simulink model "BMS_OL_Harness_advancedcell"  (R2017b)
settings: Solver=FixedStepDiscrete  StartTime=0.0  StopTime=660  FixedStep=BMSk_stepSize  RelTol=1e-3  EnableMultiTasking=on
values from neighbouring files (symbols this model uses):
  BMSk_stepSize = 0.1    [BMS_OL_init.m]
settings Model: PauseTimes=22  Creator=ms2zwt  LastModifiedBy=nctzv8
settings ConfigSet: Description=OpenECU configuration set for code generation under RTW-EC.
settings SolverCC: PositivePriorityOrder=on
settings DataIOCC: LimitDataPoints=on  SaveFormat=Array  SignalLoggingSaveFormat=ModelDataLogs
settings OptimizationCC: DefaultParameterBehavior=Inlined  InlineInvariantSignals=on  ExpressionDepthLimit=2147483647  StateBitsets=on  DataBitsets=on  ZeroExternalMemoryAtStartup=off  ZeroInternalMemoryAtStartup=off  NoFixptDivByZeroProtection=on  EfficientFloat2IntCast=on  LifeSpan=1
settings DebuggingCC: SaveWithParameterizedLinksMsg=none  UnderspecifiedInitializationDetection=Classic  MergeDetectMultiDrivingBlocksExec=none  SignalResolutionControl=TryResolveAllWithWarning  MultiTaskDSMMsg=warning  MultiTaskCondExecSysMsg=none  SingleTaskRateTransMsg=error  CheckMatrixSingularityMsg=warning  VectorMatrixConversionMsg=warning  FcnCallInpInsideContextMsg=warning  SignalLabelMismatchMsg=warning  AllowSymbolicDim=off  StateNameClashWarn=warning  SFUnexpectedBacktrackingDiag=warning  SFNoUnconditionalDefaultTransitionDiag=warning  SFExecutionAtInitializationDiag=none
settings HardwareCC: ProdBitPerPointer=32  ProdBitPerSizeT=32  ProdBitPerPtrDiffT=32  ProdLargestAtomicInteger=Long  ProdLargestAtomicFloat=Double  ProdEndianess=BigEndian  ProdWordSize=32  ProdHWDeviceType=Freescale->32-bit PowerPC  TargetIntDivRoundTo=Zero  TargetEndianess=BigEndian  TargetHWDeviceType=Freescale->32-bit PowerPC  ProdEqTarget=off
settings ModelReferenceCC: PropagateSignalLabelsOutOfModel=off
settings SFSimCC: MATLABDynamicMemAlloc=off
settings RTWCC: SystemTargetFile=openecu_ert.tlc  MakeCommand=make_rtw optimized_floating_point=1  TemplateMakefile=openecu_ert_r2015b_64.tmf  Description=OpenECU Platform Target (ERT, optimised floating-point code)  RetainRTWFile=on  IncludeHyperlinkInReport=on
settings CodeAppCC: ForceParamTrailComments=on  IgnoreCustomStorageClasses=off  SimulinkDataObjDesc=on  CustomSymbolStrType=$N$R$M  InsertBlockDesc=on  StateflowObjectComments=on  InternalIdentifier=Classic
settings STFCustomTargetCC: TargetLibSuffix=.a  GenerateSampleERTMain=on  IncludeMdlTerminateFcn=off  CombineOutputUpdateFcns=on  IncludeFileDelimiter=UseQuote  ERTCustomFileBanners=on  SupportContinuousTime=off  RemoveResetFunc=on  MATLABClassNameForMDSCustomization=Simulink.SoftwareTarget.ERTCustomization  GRTInterface=off  SystemTargetFile=openecu_ert.tlc
settings ERTTargetCC: MultiwordLength=2048  GenerateSampleERTMain=on  ParMdlRefBuildCompliant=off  CompOptLevelCompliant=off  ConcurrentExecutionCompliant=off  IncludeMdlTerminateFcn=off  IncludeFileDelimiter=UseQuote  SupportNonInlinedSFcns=on  ModelStepFunctionPrototypeControlCompliant=off  CPPClassGenCompliant=off  UseToolchainInfoCompliant=off  ExtModeMexFile=noextcomm  InlinedParameterPlacement=NonHierarchical  ERTSrcFileBannerTemplate=oe_code_c_template.cgt  ERTHdrFileBannerTemplate=oe_code_h_template.cgt  ERTDataSrcFileTemplate=oe_data_c_template.cgt  ERTDataHdrFileTemplate=oe_data_h_template.cgt  ERTCustomFileTemplate=example_file_process.tlc  GlobalDataDefinition=InSeparateSourceFile  GlobalDataReference=InSeparateHeaderFile  ConvertIfToSwitch=off  SuppressUnreachableDefaultCases=off  EnableUserReplacementTypes=on
settings ConfigComp: CovMetricSettings=dw  CovHtmlReporting=on  CovSaveCumulativeToWorkspaceVar=on  CovSaveSingleToWorkspaceVar=on  CovExternalEMLEnable=off

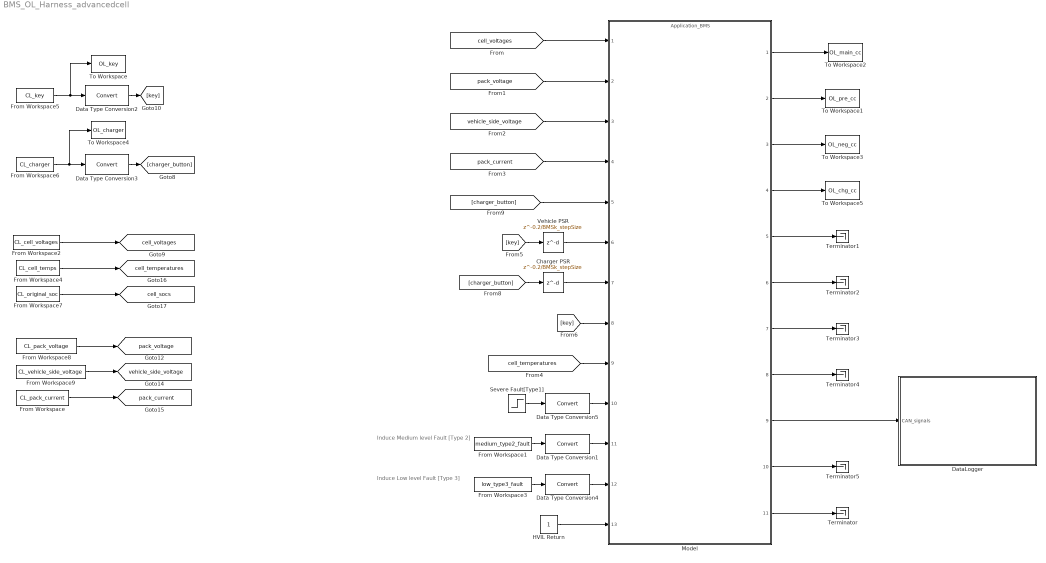
== system BMS_OL_Harness_advancedcell ==
  note: Induce Medium level Fault
      | [Type 2]
  note: Induce Low level Fault
      | [Type 3]
  Charger PSR : Delay  DelayLength=0.2/BMSk_stepSize
  Data Type Conversion{1..5} (5 alike) : DataTypeConversion
  DataLogger : Subsystem
  From Workspace : FromWorkspace  VariableName=CL_pack_current  SampleTime=BMSk_stepSize
  From Workspace1 : FromWorkspace  VariableName=medium_type2_fault  SampleTime=BMSk_stepSize
  From Workspace2 : FromWorkspace  VariableName=CL_cell_voltages  SampleTime=BMSk_stepSize
  From Workspace3 : FromWorkspace  VariableName=low_type3_fault  SampleTime=BMSk_stepSize
  From Workspace4 : FromWorkspace  VariableName=CL_cell_temps  SampleTime=BMSk_stepSize
  From Workspace5 : FromWorkspace  VariableName=CL_key  SampleTime=BMSk_stepSize
  From Workspace6 : FromWorkspace  VariableName=CL_charger  SampleTime=BMSk_stepSize
  From Workspace7 : FromWorkspace  VariableName=CL_original_soc  SampleTime=BMSk_stepSize
  From Workspace8 : FromWorkspace  VariableName=CL_pack_voltage  SampleTime=BMSk_stepSize
  From Workspace9 : FromWorkspace  VariableName=CL_vehicle_side_voltage  SampleTime=BMSk_stepSize
  HVIL Return : Constant  OutDataTypeStr=double  SampleTime=-1
  Model : ModelReference  ModelNameDialog=Application_BMS.slx  SimulationMode=Normal  ModelReferenceVersion=1.801
  Severe Fault[Type1] : Step  Time=0  After=0
  Terminator{,1..5} (6 alike) : Terminator
  To Workspace : ToWorkspace  VariableName=OL_key  SaveFormat=Timeseries  SampleTime=-1
  To Workspace1 : ToWorkspace  VariableName=OL_pre_cc  SaveFormat=Timeseries  SampleTime=-1
  To Workspace2 : ToWorkspace  VariableName=OL_main_cc  SaveFormat=Timeseries  SampleTime=-1
  To Workspace3 : ToWorkspace  VariableName=OL_neg_cc  SaveFormat=Timeseries  SampleTime=-1
  To Workspace4 : ToWorkspace  VariableName=OL_charger  SaveFormat=Timeseries  SampleTime=-1
  To Workspace5 : ToWorkspace  VariableName=OL_chg_cc  SaveFormat=Timeseries  SampleTime=-1
  Vehicle PSR : Delay  DelayLength=0.2/BMSk_stepSize
  tag scope: cell_socs=global, cell_temperatures=global, cell_voltages=global, pack_current=global, pack_voltage=global, vehicle_side_voltage=global
  wires:
  [cell_temperatures] -> Model/9
  Vehicle PSR/1 -> Model/6
  [key] -> Vehicle PSR/1
  [key] -> Model/8
  [charger_button] -> Model/5
  Charger PSR/1 -> Model/7
  [charger_button] -> Charger PSR/1
  Model/4 -> To Workspace5/1
  Model/3 -> To Workspace3/1
  Model/1 -> To Workspace2/1
  Data Type Conversion2/1 -> [key]
  Data Type Conversion4/1 -> Model/12
  From Workspace1/1 -> Data Type Conversion1/1
  Data Type Conversion5/1 -> Model/10
  [pack_current] -> Model/4
  [vehicle_side_voltage] -> Model/3
  [pack_voltage] -> Model/2
  [cell_voltages] -> Model/1
  Model/9 -> DataLogger/1(CAN_signals)
  Model/2 -> To Workspace1/1
  Data Type Conversion3/1 -> [charger_button]
  From Workspace5/1 -> To Workspace/1, Data Type Conversion2/1
  From Workspace6/1 -> To Workspace4/1, Data Type Conversion3/1
  Data Type Conversion1/1 -> Model/11
  Model/11 -> Terminator/1
  HVIL Return/1 -> Model/13
  From Workspace3/1 -> Data Type Conversion4/1
  Model/5 -> Terminator1/1
  Model/6 -> Terminator2/1
  Model/7 -> Terminator3/1
  Model/8 -> Terminator4/1
  Model/10 -> Terminator5/1
  From Workspace2/1 -> [cell_voltages]
  From Workspace4/1 -> [cell_temperatures]
  From Workspace7/1 -> [cell_socs]
  From Workspace8/1 -> [pack_voltage]
  From Workspace9/1 -> [vehicle_side_voltage]
  From Workspace/1 -> [pack_current]
  Severe Fault[Type1]/1 -> Data Type Conversion5/1

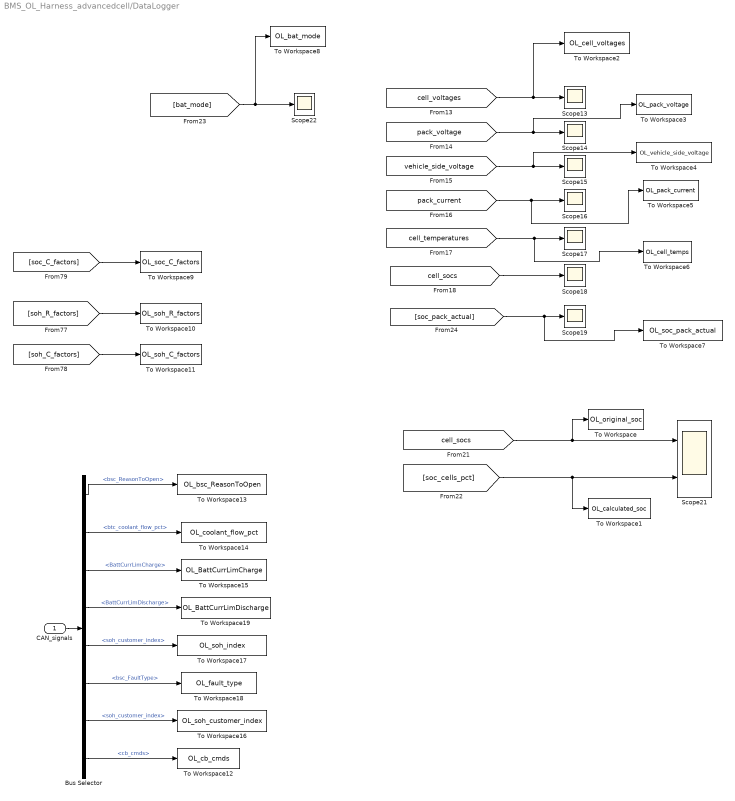
== system BMS_OL_Harness_advancedcell/DataLogger ==
  CAN_signals : Inport
  Bus Selector : BusSelector  OutputSignals=bsc_output.bsc_ReasonToOpen,btc_output.btc_coolant_flow_pct,sop_output.BattCurrLimCharge,sop_output.BattCurrLimDischarge,soh_output.soh_customer_index,bsc_output.bsc_FaultType,soh_output.soh_customer_index,cb_output.cb_cmds
  Scope{13..19,22} (8 alike) : Scope
  Scope21 : Scope  NumInputPorts=2
  To Workspace : ToWorkspace  VariableName=OL_original_soc  SaveFormat=Timeseries  SampleTime=-1
  To Workspace1 : ToWorkspace  VariableName=OL_calculated_soc  SaveFormat=Timeseries  SampleTime=-1
  To Workspace10 : ToWorkspace  VariableName=OL_soh_R_factors  SaveFormat=Timeseries  SampleTime=-1
  To Workspace11 : ToWorkspace  VariableName=OL_soh_C_factors  SaveFormat=Timeseries  SampleTime=-1
  To Workspace12 : ToWorkspace  VariableName=OL_cb_cmds  SaveFormat=Timeseries  SampleTime=-1
  To Workspace13 : ToWorkspace  VariableName=OL_bsc_ReasonToOpen  SaveFormat=Timeseries  SampleTime=-1
  To Workspace14 : ToWorkspace  VariableName=OL_coolant_flow_pct  SaveFormat=Timeseries  SampleTime=-1
  To Workspace15 : ToWorkspace  VariableName=OL_BattCurrLimCharge  SaveFormat=Timeseries  SampleTime=-1
  To Workspace16 : ToWorkspace  VariableName=OL_soh_customer_index  SaveFormat=Timeseries  SampleTime=-1
  To Workspace17 : ToWorkspace  VariableName=OL_soh_index  SaveFormat=Timeseries  SampleTime=-1
  To Workspace18 : ToWorkspace  VariableName=OL_fault_type  SaveFormat=Timeseries  SampleTime=-1
  To Workspace19 : ToWorkspace  VariableName=OL_BattCurrLimDischarge  SaveFormat=Timeseries  SampleTime=-1
  To Workspace2 : ToWorkspace  VariableName=OL_cell_voltages  SaveFormat=Timeseries  SampleTime=-1
  To Workspace3 : ToWorkspace  VariableName=OL_pack_voltage  SaveFormat=Timeseries  SampleTime=-1
  To Workspace4 : ToWorkspace  VariableName=OL_vehicle_side_voltage  SaveFormat=Timeseries  SampleTime=-1
  To Workspace5 : ToWorkspace  VariableName=OL_pack_current  SaveFormat=Timeseries  SampleTime=-1
  To Workspace6 : ToWorkspace  VariableName=OL_cell_temps  SaveFormat=Timeseries  SampleTime=-1
  To Workspace7 : ToWorkspace  VariableName=OL_soc_pack_actual  SaveFormat=Timeseries  SampleTime=-1
  To Workspace8 : ToWorkspace  VariableName=OL_bat_mode  SaveFormat=Timeseries  SampleTime=-1
  To Workspace9 : ToWorkspace  VariableName=OL_soc_C_factors  SaveFormat=Timeseries  SampleTime=-1
  wires:
  [cell_voltages] -> To Workspace2/1, Scope13/1
  [pack_voltage] -> To Workspace3/1, Scope14/1
  [vehicle_side_voltage] -> To Workspace4/1, Scope15/1
  [pack_current] -> To Workspace5/1, Scope16/1
  [cell_temperatures] -> To Workspace6/1, Scope17/1
  [cell_socs] -> Scope18/1
  [cell_socs] -> To Workspace/1, Scope21/1
  [bat_mode] -> To Workspace8/1, Scope22/1
  [soc_cells_pct] -> To Workspace1/1, Scope21/2
  [soc_pack_actual] -> To Workspace7/1, Scope19/1
  [soc_C_factors] -> To Workspace9/1
  [soh_C_factors] -> To Workspace11/1
  [soh_R_factors] -> To Workspace10/1
  CAN_signals/1 -> Bus Selector/1
  Bus Selector/1 -> To Workspace13/1  "<bsc_ReasonToOpen>"
  Bus Selector/2 -> To Workspace14/1  "<btc_coolant_flow_pct>"
  Bus Selector/3 -> To Workspace15/1  "<BattCurrLimCharge>"
  Bus Selector/7 -> To Workspace16/1  "<soh_customer_index>"
  Bus Selector/6 -> To Workspace18/1  "<bsc_FaultType>"
  Bus Selector/5 -> To Workspace17/1  "<soh_customer_index>"
  Bus Selector/4 -> To Workspace19/1  "<BattCurrLimDischarge>"
  Bus Selector/8 -> To Workspace12/1  "<cb_cmds>"
